simulink model "tetra_mod_qpsk"  (R2022a)
settings: Solver=FixedStepDiscrete  StartTime=0.0  StopTime=10  RelTol=1e-3
undefined symbols (not defined in the file): gcbh, get, rcfiltgaincompat
libraries: commseqgen3 x2, commcnvcod2 x2, commdigbbndpm3 x2, commsink2 x2, commfilt2 x2, commrandsrc2 x1, commchan3 x1, dspvision x1
settings Model: Creator=tisc1101  LastModifiedBy=Admin
settings SolverCC: AlgebraicLoopSolver=TrustRegion
settings DataIOCC: LimitDataPoints=on  SaveFormat=Array  SignalLoggingSaveFormat=ModelDataLogs  ReturnWorkspaceOutputs=off
settings OptimizationCC: ExpressionDepthLimit=2147483647  LifeSpan=inf
settings DebuggingCC: UnderspecifiedInitializationDetection=Classic  MergeDetectMultiDrivingBlocksExec=none  SolverPrmCheckMsg=warning  FcnCallInpInsideContextMsg=warning  UnconnectedInputMsg=warning  UnconnectedOutputMsg=warning  UnconnectedLineMsg=warning  StateNameClashWarn=warning  SFUnexpectedBacktrackingDiag=warning  SFNoUnconditionalDefaultTransitionDiag=warning  SFExecutionAtInitializationDiag=none  SFMachineParentedDataDiag=warning  ArithmeticOperatorsInVariantConditions=warning
settings HardwareCC: ProdBitPerPointer=32  ProdBitPerSizeT=32  ProdBitPerPtrDiffT=32  ProdLargestAtomicFloat=None  ProdIntDivRoundTo=Undefined  ProdEndianess=Unspecified  ProdWordSize=32  ProdHWDeviceType=32-bit Generic
settings ModelReferenceCC: PropagateSignalLabelsOutOfModel=off
settings SFSimCC: SimUseLocalCustomCode=off  SimParseCustomCode=off  CustomCodeUndefinedFunction=UseInterfaceOnly
settings RTWCC: RTWUseLocalCustomCode=off
settings CodeAppCC: StateflowObjectComments=on
settings GRTTargetCC: TargetLangStandard=C89/C90 (ANSI)  CombineOutputUpdateFcns=off  GRTInterface=on
settings ConfigComp: CovMetricSettings=dw  CovSaveCumulativeToWorkspaceVar=on  CovSaveSingleToWorkspaceVar=on  CovExternalEMLEnable=off

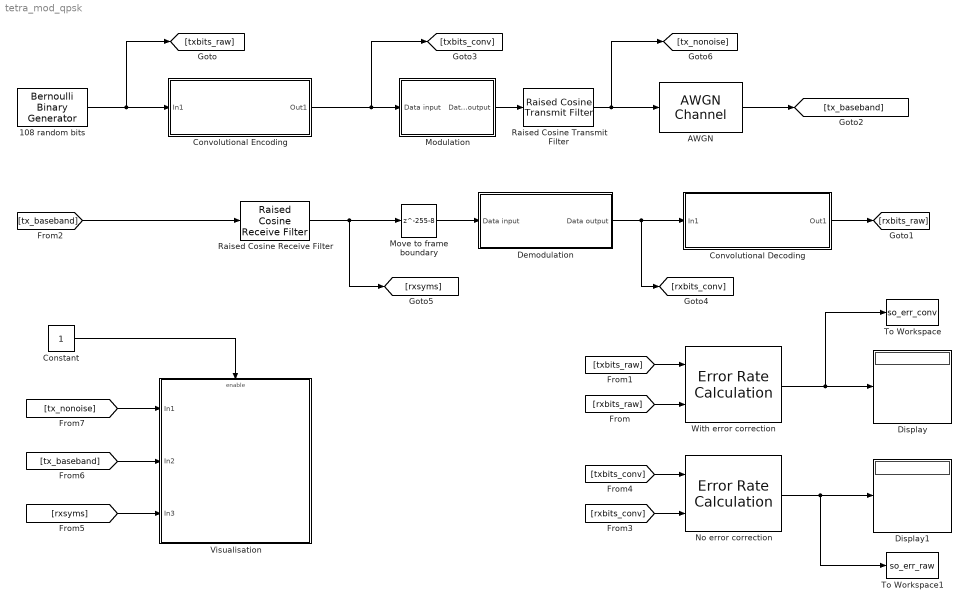
== system tetra_mod_qpsk ==
  108 random bits : commrandsrc2/Bernoulli Binary Generator  P=0.5  seed=61  Ts=1/(36000/512*108)  frameBased=on  sampPerFrame=108  orient=off  outDataType=double
      settings: SourceProductBaseCode=CM
  AWGN : commchan3/AWGN Channel  InputProcessing=Columns as channels (frame based)  seed=67  noiseMode="Signal to noise ratio  (SNR)"  EbNodB=10  EsNodB=10  SNRdB=20  bitsPerSym=1  Ps=1  Tsym=1  variance=1
  Constant : Constant
  Convolutional Decoding : Subsystem
  Convolutional Encoding : Subsystem
  Demodulation : Subsystem
  Display : Display
  Display1 : Display
  Modulation : Subsystem
  Move to frame boundary : Delay  DelayLength=255-8
  No error correction : commsink2/Error Rate Calculation  N=216  st_delay=0  cp_mode=Entire frame  subframe=[]  PMode=Port  WsName=ErrorVec  RsMode2=off  stop=off  numErr=100  maxBits=1e6
  Raised Cosine Receive Filter : commfilt2/Raised Cosine Receive Filter  filtType=Square root  R=0.35  filtSpan=2*(4)  N=8  downFactor=8  downOffset=0  filterGain=rcfiltgaincompat(gcbh)  InputProcessing=Columns as channels (frame based)  RateOptions=Enforce single-rate processing  framing=Maintain input frame rate  checkCoeff=off  variableName=rcRxFilt  currentFiltSpan=2*(4)  D=4  inputOffset=0  sampMode=Mute  saveAsFlag=0  rateMode=Downsampling  checkGain=Normalized  launchFVT=off  roundingMode=Floor  overflowMode=off  coeffDataTypeStr=Inherit: Same word length as input  coeffMin=[]  coeffMax=[]  coeffLastDataTypeStr=Inherit: Same word length as input  accumDataTypeStr=Inherit: Same as product output  accumLastDataTypeStr=Inherit: Same as product output  outputDataTypeStr=Inherit: Same as accumulator  outputMin=[]  outputMax=[]  outputLastDataTypeStr=Inherit: Same as accumulator
  Raised Cosine Transmit Filter : commfilt2/Raised Cosine Transmit Filter  filtType=Square root  R=0.35  filtSpan=2*(4)  N=8  filterGain=rcfiltgaincompat(gcbh)  InputProcessing=Columns as channels (frame based)  RateOptions=Enforce single-rate processing  framing=Maintain input frame rate  checkCoeff=off  variableName=rcTxFilt  checkGain=Normalized  sampMode=Mute  saveAsFlag=0  currentFiltSpan=2*(4)  D=4  launchFVT=off  roundingMode=Floor  overflowMode=off  coeffDataTypeStr=Inherit: Same word length as input  coeffMin=[]  coeffMax=[]  coeffLastDataTypeStr=Inherit: Same word length as input  outputDataTypeStr=Inherit: Same as accumulator  outputMin=[]  outputMax=[]  outputLastDataTypeStr=Inherit: Same as accumulator
  To Workspace : ToWorkspace  VariableName=so_err_conv  SaveFormat=Structure  SampleTime=-1
  To Workspace1 : ToWorkspace  VariableName=so_err_raw  SaveFormat=Structure  SampleTime=-1
  Visualisation : Subsystem  TreatAsAtomicUnit=on
  With error correction : commsink2/Error Rate Calculation  N=156  st_delay=0  cp_mode=Entire frame  subframe=[]  PMode=Port  WsName=ErrorVec  RsMode2=off  stop=off  numErr=100  maxBits=1e6
  wires:
  Modulation/1(Data output) -> Raised Cosine Transmit Filter/1
  Demodulation/1(Data output) -> [rxbits_conv], Convolutional Decoding/1(In1)
  [rxbits_raw] -> With error correction/2
  With error correction/1 -> Display/1, To Workspace/1
  Raised Cosine Transmit Filter/1 -> AWGN/1, [tx_nonoise]
  [tx_baseband] -> Raised Cosine Receive Filter/1
  Raised Cosine Receive Filter/1 -> Move to frame boundary/1, [rxsyms]
  Move to frame boundary/1 -> Demodulation/1(Data input)
  AWGN/1 -> [tx_baseband]
  Convolutional Encoding/1(Out1) -> Modulation/1(Data input), [txbits_conv]
  Convolutional Decoding/1(Out1) -> [rxbits_raw]
  [txbits_raw] -> With error correction/1
  [rxbits_conv] -> No error correction/2
  No error correction/1 -> Display1/1, To Workspace1/1
  [txbits_conv] -> No error correction/1
  108 random bits/1 -> Convolutional Encoding/1(In1), [txbits_raw]
  Constant/1 -> Visualisation/Enable
  [tx_baseband] -> Visualisation/2(In2)
  [rxsyms] -> Visualisation/3(In3)
  [tx_nonoise] -> Visualisation/1(In1)

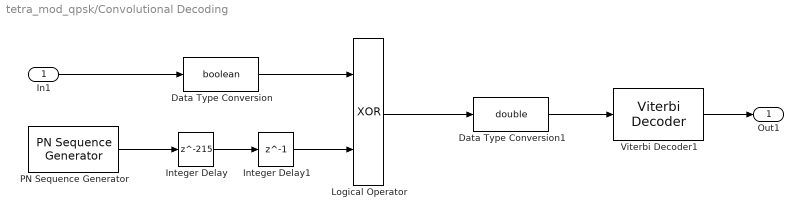
== system tetra_mod_qpsk/Convolutional Decoding ==
  In1 : Inport
  Data Type Conversion : DataTypeConversion  OutDataTypeStr=boolean  SaturateOnIntegerOverflow=off  RndMeth=Floor
  Data Type Conversion1 : DataTypeConversion  OutDataTypeStr=double  SaturateOnIntegerOverflow=off  RndMeth=Floor
  Integer Delay : Delay  DelayLength=215  InitialCondition=0
  Integer Delay1 : Delay  DelayLength=1  InitialCondition=0
  Logical Operator : Logic  Operator=XOR  AllPortsSameDT=off  OutDataTypeStr=boolean
  PN Sequence Generator : commseqgen3/PN Sequence Generator  poly=[1 1 1 0 1 1 0 1 1 0 1 1 1 0 0 0 1 0 0 0 0 0 1 1 0 0 1 0 0 0 0 0 1]  ini_sta=[0 1 0 1 0 1 0 1 0 1 0 1 0 1 0 1 0 1 0 1 0 1 0 1 0 1 0 1 0 1 1 1]  outBitMaskSource=Dialog parameter  shift=0  outVarSiz=off  maxOutSizeMode=Dialog parameter  maxOutSize=[10 1]  Ts=1/(36000/512*216)  sampPerFrame=216  reset=off  bitPackedOutputs=off  outDataType=boolean  numPackedBits=8  bitPackDataSigned=off  bitPackedOutDType=double
  Viterbi Decoder1 : commcnvcod2/Viterbi Decoder  trellis=poly2trellis(7, [171 133])  isPunctured=off  punctureVector=[1; 1; 0; 1; 0; 1]  erasures=off  dectype=Hard decision  nsdecb=3  runSigValErrCheck=off  tbdepth=48  opmode=Continuous  reset=off  delayedResetAction=off  smWordLength=16  outDataType=double
      settings: SourceProductBaseCode=CM
  Out1 : Outport
  wires:
  Viterbi Decoder1/1 -> Out1/1
  Logical Operator/1 -> Data Type Conversion1/1
  In1/1 -> Data Type Conversion/1
  PN Sequence Generator/1 -> Integer Delay/1
  Data Type Conversion/1 -> Logical Operator/1
  Data Type Conversion1/1 -> Viterbi Decoder1/1
  Integer Delay/1 -> Integer Delay1/1
  Integer Delay1/1 -> Logical Operator/2

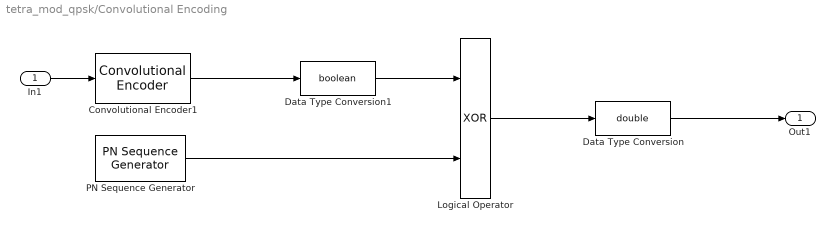
== system tetra_mod_qpsk/Convolutional Encoding ==
  In1 : Inport
  Convolutional Encoder1 : commcnvcod2/Convolutional Encoder  trellis=poly2trellis(7, [171 133])  opMode=Continuous  DelayedResetAction=off  hasIniStPort=off  hasFinStPort=off  usePuncVector=off  punctureVector=[1; 1; 0; 1; 0; 1]  reset=Unused parameter value
      settings: SourceProductBaseCode=CM
  Data Type Conversion : DataTypeConversion  OutDataTypeStr=double  SaturateOnIntegerOverflow=off  RndMeth=Floor
  Data Type Conversion1 : DataTypeConversion  OutDataTypeStr=boolean  SaturateOnIntegerOverflow=off  RndMeth=Floor
  Logical Operator : Logic  Operator=XOR  AllPortsSameDT=off  OutDataTypeStr=boolean
  PN Sequence Generator : commseqgen3/PN Sequence Generator  poly=[1 1 1 0 1 1 0 1 1 0 1 1 1 0 0 0 1 0 0 0 0 0 1 1 0 0 1 0 0 0 0 0 1]  ini_sta=[0 1 0 1 0 1 0 1 0 1 0 1 0 1 0 1 0 1 0 1 0 1 0 1 0 1 0 1 0 1 1 1]  outBitMaskSource=Dialog parameter  shift=0  outVarSiz=off  maxOutSizeMode=Dialog parameter  maxOutSize=[10 1]  Ts=1/(36000/512*216)  sampPerFrame=216  reset=off  bitPackedOutputs=off  outDataType=boolean  numPackedBits=8  bitPackDataSigned=off  bitPackedOutDType=double
  Out1 : Outport
  wires:
  In1/1 -> Convolutional Encoder1/1
  Convolutional Encoder1/1 -> Data Type Conversion1/1
  PN Sequence Generator/1 -> Logical Operator/2
  Logical Operator/1 -> Data Type Conversion/1
  Data Type Conversion/1 -> Out1/1
  Data Type Conversion1/1 -> Logical Operator/1

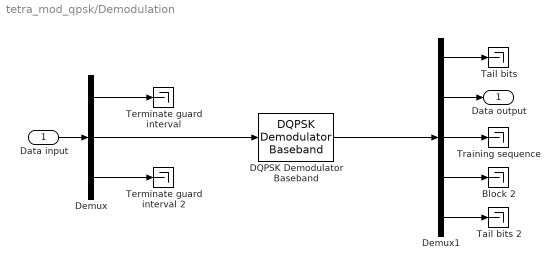
== system tetra_mod_qpsk/Demodulation ==
  Data input : Inport
  Block 2 : Terminator
  DQPSK Demodulator Baseband : commdigbbndpm3/DQPSK Demodulator Baseband  OutType=Bit  Dec=Gray  Ph=pi/4  outDtype1=Inherit via internal rule  outDtype2=Inherit via internal rule
      settings: SourceProductBaseCode=CM
  Demux : Demux  Outputs=[17 231 7]
  Demux1 : Demux  Outputs=[4 216 22 216 4]
  Tail bits : Terminator
  Tail bits 2 : Terminator
  Terminate guard interval : Terminator
  Terminate guard interval 2 : Terminator
  Training sequence : Terminator
  Data output : Outport
  wires:
  Demux/1 -> Terminate guard interval/1
  Demux/3 -> Terminate guard interval 2/1
  Demux/2 -> DQPSK Demodulator Baseband/1
  DQPSK Demodulator Baseband/1 -> Demux1/1
  Demux1/1 -> Tail bits/1
  Demux1/3 -> Training sequence/1
  Demux1/4 -> Block 2/1
  Demux1/5 -> Tail bits 2/1
  Data input/1 -> Demux/1
  Demux1/2 -> Data output/1

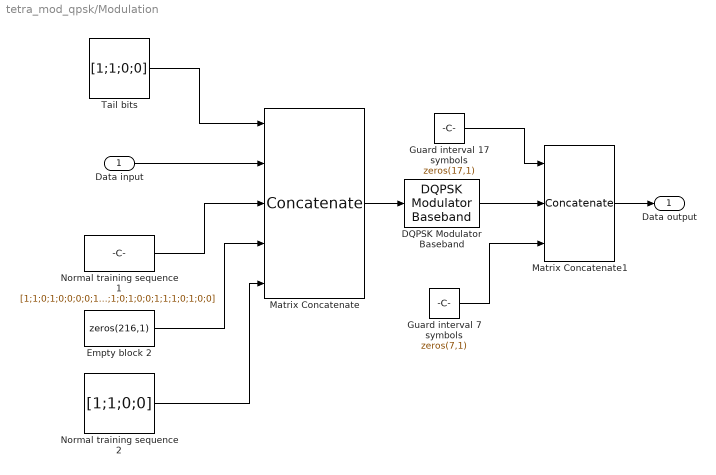
== system tetra_mod_qpsk/Modulation ==
  Data input : Inport
  DQPSK Modulator Baseband : commdigbbndpm3/DQPSK Modulator Baseband  InType=Bit  Enc=Gray  Ph=pi/4  outDtype=double
      settings: SourceProductBaseCode=CM
  Empty block 2 : Constant  Value=zeros(216,1)  VectorParams1D=off
      settings: SamplingMode=Frame based
  Guard interval 17 symbols : Constant  Value=zeros(17,1)  VectorParams1D=off
      settings: SamplingMode=Frame based
  Guard interval 7 symbols : Constant  Value=zeros(7,1)  VectorParams1D=off
      settings: SamplingMode=Frame based
  Matrix Concatenate : Concatenate  NumInputs=5  Mode=Multidimensional array
  Matrix Concatenate1 : Concatenate  NumInputs=3  Mode=Multidimensional array
  Normal training sequence 1 : Constant  Value=[1;1;0;1;0;0;0;0;1;1;1;0;1;0;0;1;1;1;0;1;0;0]  VectorParams1D=off
      settings: SamplingMode=Frame based
  Normal training sequence 2 : Constant  Value=[1;1;0;0]  VectorParams1D=off
      settings: SamplingMode=Frame based
  Tail bits : Constant  Value=[1;1;0;0]  VectorParams1D=off
      settings: SamplingMode=Frame based
  Data output : Outport
  wires:
  Tail bits/1 -> Matrix Concatenate/1
  Data input/1 -> Matrix Concatenate/2
  Normal training sequence 1/1 -> Matrix Concatenate/3
  Empty block 2/1 -> Matrix Concatenate/4
  Normal training sequence 2/1 -> Matrix Concatenate/5
  Matrix Concatenate/1 -> DQPSK Modulator Baseband/1
  Guard interval 17 symbols/1 -> Matrix Concatenate1/1
  DQPSK Modulator Baseband/1 -> Matrix Concatenate1/2
  Guard interval 7 symbols/1 -> Matrix Concatenate1/3
  Matrix Concatenate1/1 -> Data output/1

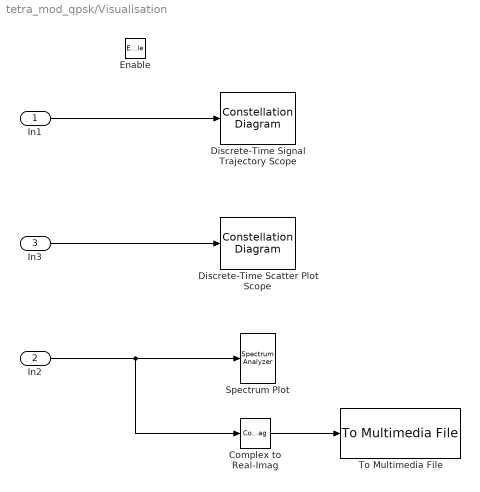
== system tetra_mod_qpsk/Visualisation ==
  In1 : Inport
  In2 : Inport  Port=2
  In3 : Inport  Port=3
  Enable : EnablePort
  Complex to Real-Imag : ComplexToRealImag  Output=Real
  Discrete-Time Scatter Plot Scope : ConstellationDiagram  Tag=ScatterPlot  FigPos=get(0,'defaultfigureposition');
  Discrete-Time Signal Trajectory Scope : ConstellationDiagram  Tag=SignalTrajectory  WindowPosition=[105.000000,181.000000,560.000000,420.000000,]  ScopeFrameLocation=window  SamplesPerSymbol=8  SymbolsToDisplaySource=on  SymbolsToDisplay=400  Title=Signal Trajectory  XLimits=0.667665055503829  YLimits=0.657178779820385  ShowTrajectory=on  ColorFading=on  FigPos=get(0,'defaultfigureposition');
  Spectrum Plot : SpectrumAnalyzer
  To Multimedia File : dspvision/To Multimedia File  outputFilename=output.wav  streamSelection=Audio only  videoCompressor=None (uncompressed)  audioCompressor=None (uncompressed)  imagePorts=Separate color signals  fileType=WAV  audioDatatype=32-bit float  fourcc=RGB  videoQuality=75  mj2000CompFactor=10
  wires:
  Complex to Real-Imag/1 -> To Multimedia File/1
  In2/1 -> Complex to Real-Imag/1, Spectrum Plot/1
  In1/1 -> Discrete-Time Signal Trajectory Scope/1
  In3/1 -> Discrete-Time Scatter Plot Scope/1
